simulink model "dem_uDAQ28LT_system"  (R2020b)
settings: Solver=VariableStepAuto  StartTime=0.0  StopTime=100  RelTol=1e-3
values from neighbouring files (symbols this model uses):
  regparams = struct    [uDAQ_variables.m]
  simparams = struct    [uDAQ_variables.m]
libraries: uDAQ28LT_lib x2
settings Model: Creator=dp  LastModifiedBy=udaq

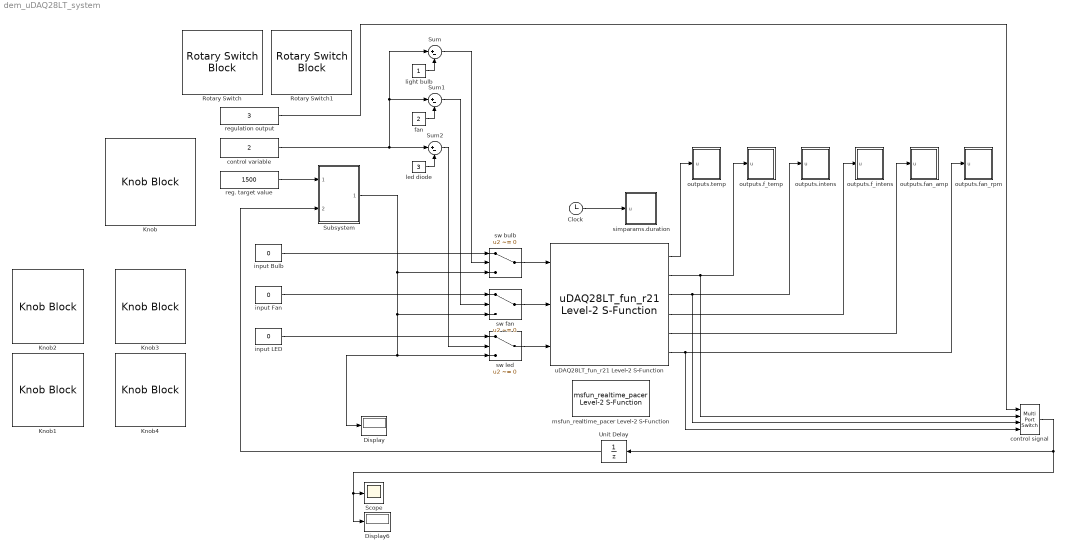
== system dem_uDAQ28LT_system ==
  Clock : Clock
  Display : Display
  Display6 : Display
  Knob : KnobBlock  ScaleMax=6000  TickInterval=500
  Knob1 : KnobBlock  ScaleMax=0.1  TickInterval=0.01
  Knob2 : KnobBlock  ScaleMax=1  TickInterval=0.1
  Knob3 : KnobBlock  TickInterval=20
  Knob4 : KnobBlock  TickInterval=20
  Rotary Switch : RotarySwitchBlock
      settings: Values={{'Bulb', 'Fan', 'LED'}, [1 2 3]}
  Rotary Switch1 : RotarySwitchBlock
      settings: Values={{'temp', 'intens', 'rpm'}, [1 2 3]}
  Scope : Scope
  Subsystem : Subsystem  mask{Kc=regparams.Kc, Ti=regparams.Ti, Umin=regparams.U_min, Umax=regparams.U_max}
      mask Display: disp('PI \nControl')
  Sum : Sum  Inputs=|+-
  Sum1 : Sum  Inputs=|+-
  Sum2 : Sum  Inputs=|+-
  Unit Delay : UnitDelay  SampleTime=simparams.Ts  HasFrameUpgradeWarning=on
  control signal : MultiPortSwitch  OutDataTypeStr=double
  control variable : Constant  Value=2  SampleTime=simparams.Ts
  fan : Constant  Value=2  SampleTime=simparams.Ts
  input Bulb : Constant  Value=0  SampleTime=simparams.Ts
  input Fan : Constant  Value=0  SampleTime=simparams.Ts
  input LED : Constant  Value=0  SampleTime=simparams.Ts
  led diode : Constant  Value=3  SampleTime=simparams.Ts
  light bulb : Constant  SampleTime=simparams.Ts
  msfun_realtime_pacer Level-2 S-Function : uDAQ28LT_lib/msfun_realtime_pacer Level-2 S-Function  simTimePerRealTime=1
  outputs.f_intens : MATLAB Function  TreatAsAtomicUnit=on  SystemSampleTime=simparams.Ts
  outputs.f_temp : MATLAB Function  TreatAsAtomicUnit=on  SystemSampleTime=simparams.Ts
  outputs.fan_amp : MATLAB Function  TreatAsAtomicUnit=on  SystemSampleTime=simparams.Ts
  outputs.fan_rpm : MATLAB Function  TreatAsAtomicUnit=on  SystemSampleTime=simparams.Ts
  outputs.intens : MATLAB Function  TreatAsAtomicUnit=on  SystemSampleTime=simparams.Ts
  outputs.temp : MATLAB Function  TreatAsAtomicUnit=on  SystemSampleTime=simparams.Ts
  reg. target value : Constant  Value=1500  OutDataTypeStr=int16  SampleTime=simparams.Ts
  regulation output : Constant  Value=3  SampleTime=simparams.Ts
  simparams.duration : MATLAB Function  TreatAsAtomicUnit=on  SystemSampleTime=simparams.Ts
  sw bulb : Switch  Criteria=u2 ~= 0  OutDataTypeStr=double
  sw fan : Switch  Criteria=u2 ~= 0  OutDataTypeStr=double
  sw led : Switch  Criteria=u2 ~= 0  OutDataTypeStr=double
  uDAQ28LT_fun_r21 Level-2 S-Function : uDAQ28LT_lib/uDAQ28LT_fun_r21 Level-2 S-Function  com=com  baud=baud  Ts=simparams.Ts
  wires:
  uDAQ28LT_fun_r21 Level-2 S-Function/1 -> outputs.temp/1(u)
  uDAQ28LT_fun_r21 Level-2 S-Function/2 -> outputs.f_temp/1(u), control signal/2
  Clock/1 -> simparams.duration/1(u)
  sw bulb/1 -> uDAQ28LT_fun_r21 Level-2 S-Function/1
  sw fan/1 -> uDAQ28LT_fun_r21 Level-2 S-Function/2
  sw led/1 -> uDAQ28LT_fun_r21 Level-2 S-Function/3
  light bulb/1 -> Sum/2
  fan/1 -> Sum1/2
  led diode/1 -> Sum2/2
  uDAQ28LT_fun_r21 Level-2 S-Function/3 -> control signal/3, outputs.intens/1(u)
  uDAQ28LT_fun_r21 Level-2 S-Function/4 -> outputs.f_intens/1(u)
  uDAQ28LT_fun_r21 Level-2 S-Function/5 -> outputs.fan_amp/1(u)
  uDAQ28LT_fun_r21 Level-2 S-Function/6 -> outputs.fan_rpm/1(u), control signal/4
  Sum/1 -> sw bulb/2
  Sum1/1 -> sw fan/2
  Sum2/1 -> sw led/2
  control variable/1 -> Sum/1, Sum1/1, Sum2/1
  input Bulb/1 -> sw bulb/1
  input Fan/1 -> sw fan/1
  input LED/1 -> sw led/1
  regulation output/1 -> control signal/1
  reg. target value/1 -> Subsystem/1(Required value)
  Subsystem/1(Control signal) -> Display/1, sw led/3, sw fan/3, sw bulb/3
  control signal/1 -> Display6/1, Scope/1, Unit Delay/1
  Unit Delay/1 -> Subsystem/2(Output)

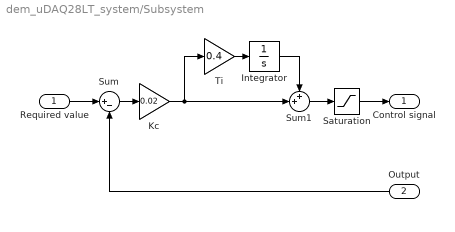
== system dem_uDAQ28LT_system/Subsystem ==
  Required value : Inport
  Output : Inport  Port=2
  Integrator : Integrator
  Kc : Gain  Gain=0.02
  Saturation : Saturate  UpperLimit=100  LowerLimit=0
  Sum : Sum  Inputs=|+-
  Sum1 : Sum  Inputs=++|
  Ti : Gain  Gain=0.4
  Control signal : Outport
  wires:
  Saturation/1 -> Control signal/1
  Required value/1 -> Sum/1
  Sum/1 -> Kc/1
  Output/1 -> Sum/2
  Kc/1 -> Ti/1, Sum1/2
  Sum1/1 -> Saturation/1
  Ti/1 -> Integrator/1
  Integrator/1 -> Sum1/1

== matlab function dem_uDAQ28LT_system/outputs.f_temp ==
  data: u input
function fcn(u)
coder.extrinsic('evalin');
evalin('base',sprintf('outputs.f_temp(end+1)=%f;',u));
end

== matlab function dem_uDAQ28LT_system/outputs.fan_amp ==
  data: u input
function fcn(u)
coder.extrinsic('evalin');
evalin('base',sprintf('outputs.fan_amp(end+1)=%f;',u));
end

== matlab function dem_uDAQ28LT_system/outputs.fan_rpm ==
  data: u input
function fcn(u)
coder.extrinsic('evalin');
evalin('base',sprintf('outputs.fan_rpm(end+1)=%f;',u));
end

== matlab function dem_uDAQ28LT_system/outputs.intens ==
  data: u input
function fcn(u)
coder.extrinsic('evalin');
evalin('base',sprintf('outputs.intens(end+1)=%f;',u));
end

== matlab function dem_uDAQ28LT_system/outputs.temp ==
  data: u input
function fcn(u)
coder.extrinsic('evalin');
evalin('base',sprintf('outputs.temp(end+1)=%f;',u));
end

== matlab function dem_uDAQ28LT_system/simparams.duration ==
  data: u input
function fcn(u)
coder.extrinsic('evalin');
evalin('base',sprintf('simparams.duration(end+1)=%f;',u));
end

== matlab function dem_uDAQ28LT_system/outputs.f_intens ==
  data: u input
function fcn(u)
coder.extrinsic('evalin');
evalin('base',sprintf('outputs.f_intens(end+1)=%f;',u));
end
